simulink model "Fei_HX_Param_estimate"  (R2025a)
settings: Solver=VariableStepAuto  StartTime=0.0  StopTime=4910  RelTol=1e-3
libraries: fl_lib x12, nesl_utility x10, SimscapeFluids_lib x4
settings Model: Creator=20112  LastModifiedBy=20112
settings DataIOCC: ReturnWorkspaceOutputsName=SDOSimTest_Log
settings SimscapeCC: SimscapeLogType=all

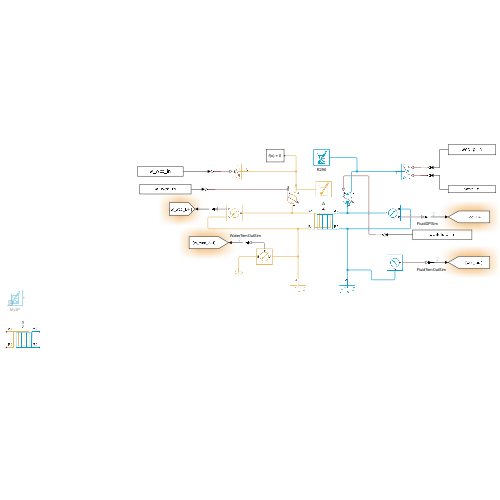
[thumbnail: Simulink's stored preview of the top-level diagram]
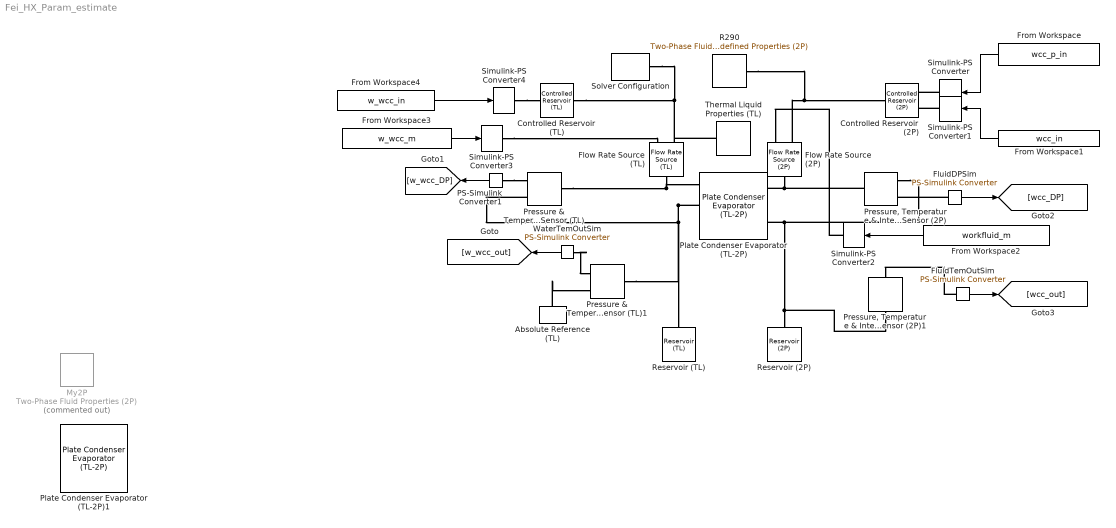
== system Fei_HX_Param_estimate ==
  Absolute Reference (TL) : fl_lib/Thermal Liquid/Elements/Absolute Reference (TL)
  Controlled Reservoir (2P) : fl_lib/Two-Phase Fluid/Elements/Controlled Reservoir (2P)  pressure_spec=foundation.enum.ControlledReservoirPressureSpec2P.Specified  energy_spec=foundation.enum.ControlledReservoirEnergySpec2P.VaporTemperature  area_A=pi/4*(11.3e-3^2) m^2  pressure_limit_spec=foundation.enum.PressureLimitSpec2P.Warn
      settings: InternalSimscapePortConfiguration="{\"Bottom\":[],\"Left\":[{\"id\":\"A\",\"label\":\"A\",\"type\":\"foundation.two_phase_fluid.two_phase_fluid\"}],\"Right\":[{\"id\":\"T\",\"label\":\"T\",\"type\":\"input\"},{\"id\":\"P\",\"label\":\"P\",\"type\":\"input\"}],\"Top\":[]}"
  Controlled Reservoir (TL) : fl_lib/Thermal Liquid/Elements/Controlled Reservoir (TL)  pressure_spec=foundation.enum.pressure_spec.atmospheric  reservoir_pressure=0.101325 MPa  area=pi/4*(35.8e-3^2) m^2
      settings: InternalSimscapePortConfiguration="{\"Bottom\":[],\"Left\":[{\"id\":\"A\",\"label\":\"A\",\"type\":\"foundation.thermal_liquid.thermal_liquid\"}],\"Right\":[{\"id\":\"T_in\",\"label\":\"T\",\"type\":\"input\"}],\"Top\":[]}"
  Flow Rate Source (2P) : fl_lib/Two-Phase Fluid/Sources/Flow Rate Source (2P)  source_type=foundation.enum.constant_controlled.controlled  flow_type=foundation.enum.mass_volumetric_flow.mass  mass_flow=0 kg/s  volumetric_flow=0 m^3/s  power_spec=foundation.enum.power_spec.none  area_A=pi/4*(11.3e-3^2) m^2  area_B=pi/4*(11.3e-3^2) m^2
      settings: InternalSimscapePortConfiguration="{\"Bottom\":[],\"Left\":[{\"id\":\"A\",\"label\":\"A\",\"type\":\"foundation.two_phase_fluid.two_phase_fluid\"},{\"id\":\"M\",\"label\":\"M\",\"type\":\"input\"}],\"Right\":[{\"id\":\"B\",\"label\":\"B\",\"type\":\"foundation.two_phase_fluid.two_phase_fluid\"}],\"Top\":[]}"
  Flow Rate Source (TL) : fl_lib/Thermal Liquid/Sources/Flow Rate Source (TL)  source_type=foundation.enum.constant_controlled.controlled  flow_type=foundation.enum.mass_volumetric_flow.volumetric  mass_flow=0 kg/s  volumetric_flow=0 m^3/s  power_spec=foundation.enum.power_spec.none  area=pi/4*(35.8e-3^2) m^2
      settings: InternalSimscapePortConfiguration="{\"Bottom\":[],\"Left\":[{\"id\":\"A\",\"label\":\"A\",\"type\":\"foundation.thermal_liquid.thermal_liquid\"},{\"id\":\"V\",\"label\":\"V\",\"type\":\"input\"}],\"Right\":[{\"id\":\"B\",\"label\":\"B\",\"type\":\"foundation.thermal_liquid.thermal_liquid\"}],\"Top\":[]}"
  FluidDPSim : nesl_utility/PS-Simulink Converter  PhysicalDomain=network_engine_domain  SubClassName=ps_output  LeftPortType=input  RightPortType=output  PseudoPeriodic=off  Frequencies=[]  VectorFormat=inherit  Unit=kPa  AffineConversion=on
  FluidTemOutSim : nesl_utility/PS-Simulink Converter  PhysicalDomain=network_engine_domain  SubClassName=ps_output  LeftPortType=input  RightPortType=output  PseudoPeriodic=off  Frequencies=[]  VectorFormat=inherit  Unit=degC  AffineConversion=on
  From Workspace : FromWorkspace  VariableName=wcc_p_in
  From Workspace1 : FromWorkspace  VariableName=wcc_in
  From Workspace2 : FromWorkspace  VariableName=workfluid_m
  From Workspace3 : FromWorkspace  VariableName=w_wcc_m
  From Workspace4 : FromWorkspace  VariableName=w_wcc_in
  My2P : fl_lib/Two-Phase Fluid/Utilities/Two-Phase Fluid Properties (2P)  Commented=on  u_min=FluidProperty.u_min kJ/kg  u_max=FluidProperty.u_max kJ/kg  p_TLU=FluidProperty.p MPa  p_crit=FluidProperty.p_crit MPa  critical_region=foundation.enum.critical_region.clip  p_crit_fraction=0.12  p_atm=0.101325 MPa  properties_range_check=simscape.enum.assert.action.error  q_rev=0.01 Pa  unorm_liq=FluidProperty.liquid.unorm  v_liq=FluidProperty.liquid.v m^3/kg  s_liq=FluidProperty.liquid.s kJ/(kg*K)  T_liq=FluidProperty.liquid.T K  nu_liq=FluidProperty.liquid.nu mm^2/s  k_liq=FluidProperty.liquid.k W/(m*K)  Pr_liq=FluidProperty.liquid.Pr  u_sat_liq=FluidProperty.liquid.u_sat kJ/kg  unorm_vap=FluidProperty.vapor.unorm  v_vap=FluidProperty.vapor.v m^3/kg  s_vap=FluidProperty.vapor.s kJ/(kg*K)  T_vap=FluidProperty.vapor.T K  nu_vap=FluidProperty.vapor.nu mm^2/s  k_vap=FluidProperty.vapor.k W/(m*K)  Pr_vap=FluidProperty.vapor.Pr  u_sat_vap=FluidProperty.vapor.u_sat kJ/kg
      settings: InternalSimscapePortConfiguration="{\"Bottom\":[],\"Left\":[],\"Right\":[{\"id\":\"A\",\"label\":\"\",\"type\":\"foundation.two_phase_fluid.two_phase_fluid\"}],\"Top\":[]}"
  PS-Simulink Converter1 : nesl_utility/PS-Simulink Converter  PhysicalDomain=network_engine_domain  SubClassName=ps_output  LeftPortType=input  RightPortType=output  PseudoPeriodic=off  Frequencies=[]  VectorFormat=inherit  Unit=kPa  AffineConversion=on
  Plate Condenser Evaporator (TL-2P) : SimscapeFluids_lib/Heat Exchangers/Two-Phase Fluid - Thermal Liquid/Plate Condenser Evaporator (TL-2P)  flow_arrangement=fluids.heat_exchangers.enum.PlateFlowArrangement.Counter  plate_num=28  plate_length=ADarcyTL m  plate_width=50e-3 m  plate_spacing=1.615e-3 m  plate_corrugation_spec=fluids.heat_exchangers.enum.PlateCorrugationSpec.EnlargementFactor  plate_enlargement_factor=1  plate_chevron_angle=60 deg  plate_depth_pitch_ratio=0.28  plate_thermal_resistance=false  plate_thermal_mass=false  plate_thickness=0.785e-3 m  plate_thermal_conductivity=15 W/(K*m)  plate_density=7800 kg/m^3  plate_specific_heat=490 J/(K*kg)  area_A1=pi/4*(35.8e-3^2) m^2  area_B1=pi/4*(35.8e-3^2) m^2  area_A2=pi/4*(11.3e-3^2) m^2  area_B2=pi/4*(11.3e-3^2) m^2  plate_pressure_loss_spec_TL=fluids.heat_exchangers.enum.PlatePressureLossSpec.Martin  plate_friction_factor_TL=49  plate_manifold_loss_coeff_TL=1.5  plate_heat_coeff_spec_TL=fluids.heat_exchangers.enum.PlateHeatCoeffSpec.Martin  plate_colburn_coeff_TL=[.141, .748, .333]  plate_martin_coeff_TL=[.122, .374, .333]  fouling_factor_TL=0 K*m^2/kW  p_init_TL=0.101325 MPa  T_init_TL=31.65 degC  plate_pressure_loss_spec_2P=fluids.heat_exchangers.enum.PlatePressureLossSpec2P.FrictionFactor  plate_friction_factor_2P=ADarcyTP  plate_manifold_loss_coeff_2P=1.5  plate_heat_coeff_spec_2P=fluids.heat_exchangers.enum.PlateHeatCoeffSpec2P.MartinLongo  plate_colburn_coeff_liq_2P=[.141, .748, .333]  plate_colburn_coeff_mix_2P=[1.875, .445, .333]  plate_colburn_coeff_vap_2P=[.141, .748, .333]  plate_martin_longo_coeff_liq_2P=[.122, .374, .333]  plate_martin_longo_coeff_mix_2P=[1.875, .445, .333]  plate_martin_longo_coeff_vap_2P=[.122, .374, .333]  fouling_factor_2P=0.2 K*m^2/kW  energy_spec_2P=foundation.enum.energy_spec.temperature  p_init_2P=1.01695 MPa  T_init_2P=31.24 degC  x_init_2P=0.5  alpha_init_2P=0.5  h_init_2P=1500 kJ/kg  u_init_2P=1500 kJ/kg
      settings: InternalSimscapePortConfiguration="{\"Bottom\":[],\"Left\":[{\"id\":\"A1\",\"label\":\"A1\",\"type\":\"foundation.thermal_liquid.thermal_liquid\"},{\"id\":\"B1\",\"label\":\"B1\",\"type\":\"foundation.thermal_liquid.thermal_liquid\"}],\"Right\":[{\"id\":\"A2\",\"label\":\"A2\",\"type\":\"foundation.two_phase_fluid.two_phase_fluid\"},{\"id\":\"B2\",\"label\":\"B2\",\"type\":\"foundation.two_phase_fluid.two_phase_fluid\"}],\"Top\":[{\"id\":\"Z\",\"label\":\"Z\",\"type\":\"output\"}]}"
  Plate Condenser Evaporator (TL-2P)1 : SimscapeFluids_lib/Heat Exchangers/Two-Phase Fluid - Thermal Liquid/Plate Condenser Evaporator (TL-2P)  flow_arrangement=fluids.heat_exchangers.enum.PlateFlowArrangement.Counter  plate_num=25  plate_length=1 m  plate_width=0.5 m  plate_spacing=5e-3 m  plate_corrugation_spec=fluids.heat_exchangers.enum.PlateCorrugationSpec.EnlargementFactor  plate_enlargement_factor=1.17  plate_chevron_angle=60 deg  plate_depth_pitch_ratio=0.28  plate_thermal_resistance=false  plate_thermal_mass=false  plate_thickness=5e-4 m  plate_thermal_conductivity=15 W/(K*m)  plate_density=7800 kg/m^3  plate_specific_heat=490 J/(K*kg)  area_A1=0.01 m^2  area_B1=0.01 m^2  area_A2=0.01 m^2  area_B2=0.01 m^2  plate_pressure_loss_spec_TL=fluids.heat_exchangers.enum.PlatePressureLossSpec.Martin  plate_friction_factor_TL=1.7  plate_manifold_loss_coeff_TL=1.5  plate_heat_coeff_spec_TL=fluids.heat_exchangers.enum.PlateHeatCoeffSpec.Martin  plate_colburn_coeff_TL=[.141, .748, .333]  plate_martin_coeff_TL=[.122, .374, .333]  fouling_factor_TL=0.1 K*m^2/kW  p_init_TL=0.101325 MPa  T_init_TL=293.15 K  plate_pressure_loss_spec_2P=fluids.heat_exchangers.enum.PlatePressureLossSpec2P.Martin  plate_friction_factor_2P=1.7  plate_manifold_loss_coeff_2P=1.5  plate_heat_coeff_spec_2P=fluids.heat_exchangers.enum.PlateHeatCoeffSpec2P.Colburn  plate_colburn_coeff_liq_2P=[.141, .748, .333]  plate_colburn_coeff_mix_2P=[1.875, .445, .333]  plate_colburn_coeff_vap_2P=[.141, .748, .333]  plate_martin_longo_coeff_liq_2P=[.122, .374, .333]  plate_martin_longo_coeff_mix_2P=[1.875, .445, .333]  plate_martin_longo_coeff_vap_2P=[.122, .374, .333]  fouling_factor_2P=0.1 K*m^2/kW  energy_spec_2P=foundation.enum.energy_spec.temperature  p_init_2P=0.101325 MPa  T_init_2P=293.15 K  x_init_2P=0.5  alpha_init_2P=0.5  h_init_2P=1500 kJ/kg  u_init_2P=1500 kJ/kg
      settings: InternalSimscapePortConfiguration="{\"Bottom\":[],\"Left\":[{\"id\":\"A1\",\"label\":\"A1\",\"type\":\"foundation.thermal_liquid.thermal_liquid\"},{\"id\":\"B1\",\"label\":\"B1\",\"type\":\"foundation.thermal_liquid.thermal_liquid\"}],\"Right\":[{\"id\":\"A2\",\"label\":\"A2\",\"type\":\"foundation.two_phase_fluid.two_phase_fluid\"},{\"id\":\"B2\",\"label\":\"B2\",\"type\":\"foundation.two_phase_fluid.two_phase_fluid\"}],\"Top\":[{\"id\":\"Z\",\"label\":\"Z\",\"type\":\"output\"}]}"
  Pressure & Temperature Sensor (TL) : fl_lib/Thermal Liquid/Sensors/Pressure & Temperature Sensor (TL)  reference=foundation.enum.MeasurementReference.difference  pressure=true  pressure_spec=foundation.enum.PressureMeasementSpec.Absolute  temperature=false
      settings: InternalSimscapePortConfiguration="{\"Bottom\":[],\"Left\":[{\"id\":\"A\",\"label\":\"A\",\"type\":\"foundation.thermal_liquid.thermal_liquid\"}],\"Right\":[{\"id\":\"B\",\"label\":\"B\",\"type\":\"foundation.thermal_liquid.thermal_liquid\"},{\"id\":\"P\",\"label\":\"P\",\"type\":\"output\"}],\"Top\":[]}"
  Pressure & Temperature Sensor (TL)1 : fl_lib/Thermal Liquid/Sensors/Pressure & Temperature Sensor (TL)  reference=foundation.enum.MeasurementReference.difference  pressure=false  pressure_spec=foundation.enum.PressureMeasementSpec.Absolute  temperature=true
      settings: InternalSimscapePortConfiguration="{\"Bottom\":[{\"id\":\"T\",\"label\":\"T\",\"type\":\"output\"}],\"Left\":[{\"id\":\"A\",\"label\":\"A\",\"type\":\"foundation.thermal_liquid.thermal_liquid\"}],\"Right\":[{\"id\":\"B\",\"label\":\"B\",\"type\":\"foundation.thermal_liquid.thermal_liquid\"}],\"Top\":[]}"
  "Pressure, Temperature & Internal Energy Sensor (2P)" : fl_lib/Two-Phase Fluid/Sensors/Pressure, Temperature & Internal Energy Sensor (2P)  reference=foundation.enum.MeasurementReference.difference  pressure=true  pressure_spec=foundation.enum.PressureMeasementSpec.Absolute  temperature=false  internal_energy=false
      settings: InternalSimscapePortConfiguration="{\"Bottom\":[],\"Left\":[{\"id\":\"A\",\"label\":\"A\",\"type\":\"foundation.two_phase_fluid.two_phase_fluid\"}],\"Right\":[{\"id\":\"B\",\"label\":\"B\",\"type\":\"foundation.two_phase_fluid.two_phase_fluid\"},{\"id\":\"P\",\"label\":\"P\",\"type\":\"output\"}],\"Top\":[]}"
  "Pressure, Temperature & Internal Energy Sensor (2P)1" : fl_lib/Two-Phase Fluid/Sensors/Pressure, Temperature & Internal Energy Sensor (2P)  reference=foundation.enum.MeasurementReference.absolute  pressure=false  pressure_spec=foundation.enum.PressureMeasementSpec.Absolute  temperature=true  internal_energy=false
      settings: InternalSimscapePortConfiguration="{\"Bottom\":[{\"id\":\"T\",\"label\":\"T\",\"type\":\"output\"}],\"Left\":[{\"id\":\"A\",\"label\":\"A\",\"type\":\"foundation.two_phase_fluid.two_phase_fluid\"}],\"Right\":[],\"Top\":[]}"
  R290 : SimscapeFluids_lib/Two-Phase Fluid/Utilities/Two-Phase Fluid Predefined Properties (2P)  fluid=fluids.two_phase_fluid.utilities.enum.Fluid.Propane  p_atm=0.101325 MPa  properties_range_check=simscape.enum.assert.action.error  q_rev=0.01 Pa
  Reservoir (2P) : fl_lib/Two-Phase Fluid/Elements/Reservoir (2P)  pressure_spec=foundation.enum.ReservoirPressureSpec2P.Specified  reservoir_pressure=1 MPa  reservoir_condensing_temperature=373.15 K  reservoir_evaporating_temperature=373.15 K  energy_spec=foundation.enum.ReservoirEnergySpec2P.Temperature  reservoir_temperature=31 degC  reservoir_quality=0.5  reservoir_void_fraction=0.5  reservoir_enthalpy=1500 kJ/kg  reservoir_internal_energy=1500 kJ/kg  reservoir_subcooling=5 deltaK  reservoir_superheating=5 deltaK  area_A=pi/4*(11.3e-3^2) m^2
  Reservoir (TL) : fl_lib/Thermal Liquid/Elements/Reservoir (TL)  pressure_spec=foundation.enum.pressure_spec.atmospheric  reservoir_pressure=0.101325 MPa  reservoir_temperature=40 degC  area=pi/4*(35.8e-3^2) m^2
  Simulink-PS Converter : nesl_utility/Simulink-PS Converter  PhysicalDomain=network_engine_domain  SubClassName=ps_input  LeftPortType=input  RightPortType=output  PseudoPeriodic=off  Frequencies=[]  NoiseDistribution=none  NoiseParameters=[]  Unit=kPa  AffineConversion=on  FilteringAndDerivatives=provide  SimscapeFilterOrder=1  InputFilterTimeConstant=0.001  UdotUserProvided=0
  Simulink-PS Converter1 : nesl_utility/Simulink-PS Converter  PhysicalDomain=network_engine_domain  SubClassName=ps_input  LeftPortType=input  RightPortType=output  PseudoPeriodic=off  Frequencies=[]  NoiseDistribution=none  NoiseParameters=[]  Unit=degC  AffineConversion=on  FilteringAndDerivatives=provide  SimscapeFilterOrder=1  InputFilterTimeConstant=0.001  UdotUserProvided=0
  Simulink-PS Converter2 : nesl_utility/Simulink-PS Converter  PhysicalDomain=network_engine_domain  SubClassName=ps_input  LeftPortType=input  RightPortType=output  PseudoPeriodic=off  Frequencies=[]  NoiseDistribution=none  NoiseParameters=[]  Unit=kg/s  AffineConversion=on  FilteringAndDerivatives=provide  SimscapeFilterOrder=1  InputFilterTimeConstant=0.001  UdotUserProvided=0
  Simulink-PS Converter3 : nesl_utility/Simulink-PS Converter  PhysicalDomain=network_engine_domain  SubClassName=ps_input  LeftPortType=input  RightPortType=output  PseudoPeriodic=off  Frequencies=[]  NoiseDistribution=none  NoiseParameters=[]  Unit=m^3/s  AffineConversion=off  FilteringAndDerivatives=provide  SimscapeFilterOrder=1  InputFilterTimeConstant=0.001  UdotUserProvided=0
  Simulink-PS Converter4 : nesl_utility/Simulink-PS Converter  PhysicalDomain=network_engine_domain  SubClassName=ps_input  LeftPortType=input  RightPortType=output  PseudoPeriodic=off  Frequencies=[]  NoiseDistribution=none  NoiseParameters=[]  Unit=degC  AffineConversion=on  FilteringAndDerivatives=provide  SimscapeFilterOrder=1  InputFilterTimeConstant=0.001  UdotUserProvided=0
  Solver Configuration : nesl_utility/Solver Configuration  PhysicalDomain=network_engine_domain  SubClassName=solver  LeftPortType=input  RightPortType=generic  Tones=[]  Harmonics=[]  SimulateNoise=off  Profile=off  UseLocalSampling=off  EnableSwitchedLinearOptims=on  FrequencyDomain=off  UseCCode=off  RelTol=0.001  AbsTol=0.001  MinStep=1e-09  ToWorkspace=off  RevertToSquareIcSolve=off  NumHomotopyIterations=100  PhasorMode=off  PhasorModeNumHarmonics=1  ConsistencySolver=NEWTON_XTOL_AFTER_FTOL  IndexReductionMethod=DerivativeReplacement  DoDC=off  ResidualTolerance=1e-09  ConsistencyTolSource=GLOBAL  ConsistencyAbsTol=0.001  ConsistencyRelTol=0.001  ConsistencyTolFactor=0.001  UseLocalSolver=off  LocalSolverChoice=NE_BACKWARD_EULER_ADVANCER  ResolveIndetEquations=on  FunctionEvalNumThread=1  LocalSolverSampleTime=0.001  DoFixedCost=off  MaxNonlinIter=3  MaxModeIter=2  ComputeImpulses=off  ImpulseIterations=2  LinearAlgebra=auto  LinearAlgebraNumThread=0  EquationFormulation=NE_TIME_EF  DelaysMemoryBudget=1024  AutomaticFiltering=on  FilteringTimeConstant=0.001  PartitionStorageMethod=AS_NEEDED  PartitionMemoryBudget=1024  PartitionMethod=ROBUST  MultibodyUseLocalSolver=off  MultibodyLocalSolverChoice=ODE1  MultibodyLocalSolverSampleTime=0.001
  Thermal Liquid Properties (TL) : SimscapeFluids_lib/Thermal Liquid/Utilities/Thermal Liquid Properties (TL)  fluid_list=fluids.thermal_liquid.utilities.enum.thermal_liquid_fluid_list.ethylene_glycol  concentration_param_EG=fluids.thermal_liquid.utilities.enum.thermal_liquid_concentration.volume_fraction  concentration_param_PG=fluids.thermal_liquid.utilities.enum.thermal_liquid_concentration.volume_fraction  c_mass_SW=3.5e-3  c_mass_EG=0.62  c_mass_PG=0.1  c_mass_GL=0.1  c_vol_EG=0.5  c_vol_PG=0.1  beta_const_EG=2.1791 GPa  beta_const_PG=2.1791 GPa  beta_const_GL=2.1791 GPa  p_min_EG=0.01 MPa  p_min_PG=0.01 MPa  p_min_GL=0.01 MPa  p_max_EG=50 MPa  p_max_PG=50 MPa  p_max_GL=50 MPa  p_atm=0.101325 MPa  properties_range_check=simscape.enum.assert.action.error
  WaterTemOutSim : nesl_utility/PS-Simulink Converter  PhysicalDomain=network_engine_domain  SubClassName=ps_output  LeftPortType=input  RightPortType=output  PseudoPeriodic=off  Frequencies=[]  VectorFormat=inherit  Unit=degC  AffineConversion=on
  wires:
  From Workspace/1 -> Simulink-PS Converter/1
  From Workspace1/1 -> Simulink-PS Converter1/1
  From Workspace2/1 -> Simulink-PS Converter2/1
  From Workspace3/1 -> Simulink-PS Converter3/1
  From Workspace4/1 -> Simulink-PS Converter4/1
  WaterTemOutSim/1 -> [w_wcc_out]
  PS-Simulink Converter1/1 -> [w_wcc_DP]
  FluidDPSim/1 -> [wcc_DP]
  FluidTemOutSim/1 -> [wcc_out]
  connections:
  Controlled Reservoir (TL)/LConn1 -- Thermal Liquid Properties (TL)/RConn1 -- Flow Rate Source (TL)/LConn1 -- Solver Configuration/RConn1
  Plate Condenser Evaporator (TL-2P)/LConn2 -- Pressure & Temperature Sensor (TL)1/LConn1 -- Reservoir (TL)/LConn1 -- Pressure & Temperature Sensor (TL)/RConn1
  Flow Rate Source (2P)/LConn1 -- R290/RConn1 -- Controlled Reservoir (2P)/LConn1
  Simulink-PS Converter/RConn1 -- Controlled Reservoir (2P)/RConn2
  Simulink-PS Converter1/RConn1 -- Controlled Reservoir (2P)/RConn1
  Simulink-PS Converter2/RConn1 -- Flow Rate Source (2P)/LConn2
  Simulink-PS Converter4/RConn1 -- Controlled Reservoir (TL)/RConn1
  Absolute Reference (TL)/LConn1 -- Pressure & Temperature Sensor (TL)1/RConn1
  WaterTemOutSim/LConn1 -- Pressure & Temperature Sensor (TL)1/RConn2
  PS-Simulink Converter1/LConn1 -- Pressure & Temperature Sensor (TL)/RConn2
  FluidDPSim/LConn1 -- "Pressure, Temperature & Internal Energy Sensor (2P)"/RConn2
  FluidTemOutSim/LConn1 -- "Pressure, Temperature & Internal Energy Sensor (2P)1"/RConn1
  "Pressure, Temperature & Internal Energy Sensor (2P)"/RConn1 -- Plate Condenser Evaporator (TL-2P)/RConn2 -- "Pressure, Temperature & Internal Energy Sensor (2P)1"/LConn1 -- Reservoir (2P)/LConn1
  Flow Rate Source (2P)/RConn1 -- "Pressure, Temperature & Internal Energy Sensor (2P)"/LConn1 -- Plate Condenser Evaporator (TL-2P)/RConn1
  Pressure & Temperature Sensor (TL)/LConn1 -- Plate Condenser Evaporator (TL-2P)/LConn1 -- Flow Rate Source (TL)/RConn1
  Simulink-PS Converter3/RConn1 -- Flow Rate Source (TL)/LConn2
